simulink model "IFSSIM_Aero"  (R2025b)
settings: Solver=FixedStepDiscrete  StartTime=0  StopTime=inf  FixedStep=1/960  RelTol=1e-3
undefined symbols (not defined in the file or in its folder): IFSSIM_abal, IFSSIM_aF, IFSSIM_bR, IFSSIM_CdA, IFSSIM_ClA, IFSSIM_hcop, IFSSIM_rho
settings Model: Creator=raulmoran  LastModifiedBy=raulmoran

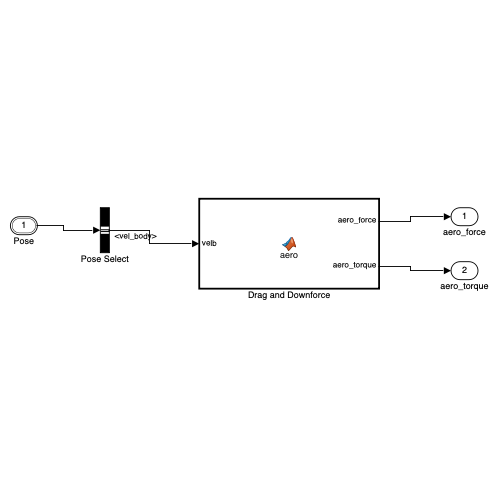
[thumbnail: Simulink's stored preview of the top-level diagram]
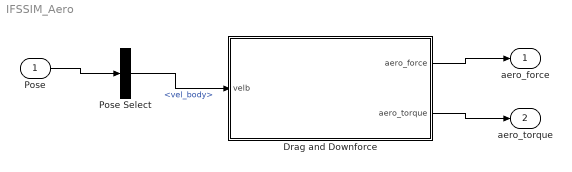
== system IFSSIM_Aero ==
  Pose : Inport  OutDataTypeStr=Bus: IFSSIM_PoseBus  BusOutputAsStruct=on
  Drag and Downforce : MATLAB Function  TreatAsAtomicUnit=on
  Pose Select : BusSelector  OutputSignals=vel_body
  aero_force : Outport  PortDimensions=3
  aero_torque : Outport  Port=2  PortDimensions=3
  wires:
  Pose/1 -> Pose Select/1
  Pose Select/1 -> Drag and Downforce/1(velb)  "<vel_body>"
  Drag and Downforce/1(aero_force) -> aero_force/1
  Drag and Downforce/2(aero_torque) -> aero_torque/1

== matlab function IFSSIM_Aero/Drag and Downforce ==
  data: velb input size=3; aero_force output size=3; aero_torque output size=3; IFSSIM_rho parameter size=1; IFSSIM_CdA parameter size=1; IFSSIM_ClA parameter size=1; IFSSIM_abal parameter size=1; IFSSIM_aF parameter size=1; IFSSIM_bR parameter size=1; IFSSIM_hcop parameter size=1
function [aero_force, aero_torque] = aero(velb, IFSSIM_rho, IFSSIM_CdA, IFSSIM_ClA, IFSSIM_abal, IFSSIM_aF, IFSSIM_bR, IFSSIM_hcop)
%#codegen
% Drag and downforce in the BODY frame.

v = norm(velb);
q = 0.5 * IFSSIM_rho * v * v;          % dynamic pressure, Pa

% Drag opposes the airflow, so it acts along -velocity. Computing it in the
% body frame means a sideways-sliding car is dragged sideways too, which is
% what actually happens and is missed by any model that only drags along x.
if v > 0.1
    drag = -q * IFSSIM_CdA * (velb / v);
else
    drag = [0; 0; 0];
end

% Downforce along BODY -Z: normal to the floor, so it rolls and pitches with
% the car rather than staying vertical in the world.
Fz_total = q * IFSSIM_ClA;
Ff = Fz_total * IFSSIM_abal;           % front
Fr = Fz_total * (1 - IFSSIM_abal);     % rear

aero_force = drag + [0; 0; -Fz_total];

% Pitch couple from the front/rear split. Application points are the axle
% positions from the CoG, so the arm tracks the wheelbase in settings.json
% rather than being a hardcoded number in the wrong unit.
Mf = cross([ IFSSIM_aF; 0; 0], [0; 0; -Ff]);
Mr = cross([-IFSSIM_bR; 0; 0], [0; 0; -Fr]);

% Drag acting above the CoG adds its own pitch couple. hcop defaults to 0 —
% no measurement, so no invented moment.
Md = cross([0; 0; IFSSIM_hcop], drag);

aero_torque = Mf + Mr + Md;
end
